simulink model "MCity_cs_withAEBSBlock"  (R2017a)
settings: Solver=ode5  StartTime=0.0  StopTime=3.95  FixedStep=1/200  RelTol=1e-3
PreLoadFcn:
  | check_NUTS_defined;
  | 
  | assignin('base',['model_closed_' bdroot],false);
InitFcn:
  | PreScanExperimentInitFcn(bdroot)
StopFcn:
  | PreScanExperimentStopFcn(bdroot)
model workspace (MAT data in the model file):
  mbox_table : struct (value not decoded)
  model_closed = 0
  sim_status = 0
values from neighbouring files (symbols this model uses):
  d_offset = -18.15    [monocityTestLeftTurn.mat]    (also in simulation_leftTurn_PreScan.m = dl/vl*vh - 43 + R)
undefined symbols (not defined in the file or in its folder): DiscIntNeverNeededParam, warningInitialVelocity, x0
libraries: simulink x78, PreScanSimulinkLibrary x14, simulink_extras x10, PreScanUsefulBlocks x4
(part 12 of 12)

== matlab function MCity_cs_withAEBSBlock/BMW_Z3_1/Subsystem/PreBraking Model/Straight road segment/Relative velocity1/Translation ==
  data: v input; xpd input; xp_dot output; TISdet parameter
function xp_dot = trans(v, xpd, TISdet)
%#codegen
%Translation of the value

xp_dot = xpd;
for i = 1 : TISdet(1)
    if xpd(i) == v
        xp_dot(i) = 0;
    end
end
end

== matlab function MCity_cs_withAEBSBlock/BMW_Z3_1/Subsystem/PreBraking Model/Straight road segment/Relative velocity1/Embedded MATLAB Function1 ==
  settings: updateMethod=DISCRETE
  data: r input; yp2 output; yp1 input; K1 input; K2 output; TISdet parameter; TISMaxRange parameter
function [yp2, K2] = modif(r, yp1, K1, TISdet, TISMaxRange)
%#codegen
% Interpolating yp value.

K2 = K1;
yp2 = yp1;

d = 50;

% Adding point
for i = 1 : TISdet(1)
   if r(i) ~= TISMaxRange(1)
      K2(i,1:d-1) = K2(i,2:d);
      K2(i,d) = yp1(i);
   end
end

% Choosing what to take
for i = 1 : TISdet(1)
    s = 0;
    suma = 0;
    for j = 1 : 50
        if K2(i,j) ~= 0
            suma = suma + K2(i,j);
            s = s + 1;
        end
    end
    yp2(i) = suma/s;
end

% Returning, if object is not detected
for i = 1: TISdet(1)
    if r(i) == TISMaxRange(1) && yp1(i) == 0
        K2(i,:,:) = zeros(d,1);
        yp2(i) = 0;
    end    
end

== matlab function MCity_cs_withAEBSBlock/Audi_A8_1/PathFollower_Preview_1/LateralController/Calculate delta steering error/eml_delta_steering_error ==
  data: v_x_vehicle input; v_x_vehicle_Min input; t_Preview_LatCtrl input; delta_steeringwheeltotal output; v_y_vehicle input; yawrate_vehicle input; CorneringStiffness_Tyres_Front input; CorneringStiffness_Tyres_Rear input; m_vehicle_total input; inertia_z_vehicle_total input; e_Lat input size=10; Pos_x_CoG_Vehicle input; wheelbase input; RefreshCounter parameter
function delta_steeringwheeltotal = eml_delta_steering_error(v_x_vehicle,v_x_vehicle_Min,t_Preview_LatCtrl,v_y_vehicle,yawrate_vehicle,CorneringStiffness_Tyres_Front,CorneringStiffness_Tyres_Rear,m_vehicle_total,inertia_z_vehicle_total,e_Lat,Pos_x_CoG_Vehicle,wheelbase,RefreshCounter)

delta_steeringwheeltotal = emlfcn_delta_steering_error(v_x_vehicle,v_x_vehicle_Min,t_Preview_LatCtrl,v_y_vehicle,yawrate_vehicle,CorneringStiffness_Tyres_Front,CorneringStiffness_Tyres_Rear,m_vehicle_total,inertia_z_vehicle_total,e_Lat,Pos_x_CoG_Vehicle,wheelbase,RefreshCounter);

% end function

== matlab function MCity_cs_withAEBSBlock/BMW_Z3_1/Subsystem/PreBraking Model/Straight road segment/Relative velocity2/Embedded MATLAB Function1 ==
  data: r input; yp2 output; yp1 input; K1 input; K2 output; TISdet parameter; TISMaxRange parameter
function [yp2, K2] = modif(r, yp1, K1, TISdet, TISMaxRange)
%#codegen
% Interpolating yp value.

K2 = K1;
yp2 = yp1;

d = 50;

% Adding point
for i = 1 : TISdet(2)
   if r(i) ~= 5*TISMaxRange(2) 
      K2(i,1:d-1) = K2(i,2:d);
      K2(i,d) = yp1(i);
   end
end

% Choosing what to take
for i = 1 : TISdet(2)
    s = 0;
    suma = 0;
    for j = 1 : 50
        if K2(i,j) ~= 0
            suma = suma + K2(i,j);
            s = s + 1;
        end
    end
    yp2(i) = suma/s;
end

% Returning, if object is not detected
for i = 1: TISdet(2)
    if r(i) == 30 && yp1(i) == 0
        K2(i,:,:) = zeros(d,1);
        yp2(i) = 0;
    end    
end

== matlab function MCity_cs_withAEBSBlock/BMW_Z3_1/Subsystem/PreBraking Model/Straight road segment/Relative velocity2/Translation ==
  data: v input; xpd input; xp_dot output; TISdet parameter
function xp_dot = trans(v, xpd, TISdet)
%#codegen
%Translation of the value

xp_dot = xpd;
for i = 1 : TISdet(2)
    if xpd(i) == v
        xp_dot(i) =0;
    end
end
end

== matlab function MCity_cs_withAEBSBlock/BMW_Z3_1/Subsystem/PreBraking Model/TIS1sorting_fun/Embedded MATLAB Function ==
  data: range input; indx input; RANGE output; TISdet parameter
function RANGE = dis(range, indx, TISdet)
%#codegen

RANGE = zeros(TISdet(1),1);
for i = 1 : length(indx)
    if indx(i) ~= 0
        RANGE(i) = range(indx(i));
    else
        RANGE(i) = 0;
    end
end

== matlab function MCity_cs_withAEBSBlock/BMW_Z3_1/Subsystem/PreBraking Model/Straight road segment/THETA Derivative1/Deriv correction ==
  data: th input; thp input; thd input; th_dot output; TISdet parameter
function th_dot = stopping(th, thp, thd, TISdet)
%#codegen
% Stopping if nothing is detected.

th_dot = thd;
for i = 1 : TISdet(2)
    if (th(i)==0 && thp(i)~=0) || (th(i)~=0 && thp(i)==0)
        th_dot(i) = 0;
    end
end
end

== matlab function MCity_cs_withAEBSBlock/BMW_Z3_1/Subsystem/PreBraking Model/Straight road segment/THETA Derivative2/Deriv correction ==
  data: th input; thp input; thd input; th_dot output; TISdet parameter
function th_dot = stopping(th, thp, thd, TISdet)
%#codegen
% Stopping if nothing is detected.

th_dot = thd;
for i = 1 : TISdet(1)
    if (th(i)==0 && thp(i)~=0) || (th(i)~=0 && thp(i)==0)
        th_dot(i) = 0;
    end
end
end

== matlab function MCity_cs_withAEBSBlock/BMW_Z3_1/Subsystem/PreBraking Model/Straight road segment/THETA Derivative2/Theta extrapolation ==
  data: r input; th1 input; th2 output; thd input; time input; K1 input; K2 output; TISdet parameter; TISMaxRange parameter
function [th2, K2] = modif(r, th1, thd, time, K1, TISdet, TISMaxRange)
%#codegen
% Interpolating theta value.

K2 = K1;
th2 = th1;

d = 10;

% Finding points used in interpolation/extrapolation.
for i = 1 : TISdet(1)
    if thd(i) ~= 0
        K2(i,1:d-1,:) = K2(i,2:d,:);
        K2(i,  d,1) = time;
        K2(i,  d,2) = th1(i);
    end
end

% Extrapolation
for i = 1 : TISdet(1)
    j = 1;
    while j < d+1 && K2(i,j,1) == 0
        j = j + 1;
    end
    
    if j > d-2
        th2(i) = th1(i);
    else
        th2(i) = interp1(K2(i,d-2:d,1),K2(i,d-2:d,2),time,'linear','extrap');
    end
end

% Returning, if object is not detected
for i = 1: TISdet(1)
    if r(i) == TISMaxRange(1) && th1(i) == 0
        K2(i,:,:) = zeros(d,2);
        th2(i) = 0;
    end    
end

end

== matlab function MCity_cs_withAEBSBlock/BMW_Z3_1/Subsystem/PreBraking Model/Straight road segment/THETA Derivative1/Theta extrapolation ==
  data: r input; th1 input; th2 output; thd input; time input; K1 input; K2 output; TISdet parameter; TISMaxRange parameter
function [th2, K2] = modif(r, th1, thd, time, K1, TISdet, TISMaxRange)
%#codegen
% Interpolating theta value.

K2 = K1;
th2 = th1;

d = 10;

% Finding points used in interpolation/extrapolation.
for i = 1 : TISdet(2)
    if thd(i) ~= 0
        K2(i,1:d-1,:) = K2(i,2:d,:);
        K2(i,  d,1) = time;
        K2(i,  d,2) = th1(i);
    end
end

% Extrapolation
for i = 1 : TISdet(2)
    j = 1;
    while j < d+1 && K2(i,j,1) == 0
        j = j + 1;
    end
    
    if j > d-2
        th2(i) = th1(i);
    else
        th2(i) = interp1(K2(i,d-2:d,1),K2(i,d-2:d,2),time,'linear','extrap');
    end
end

% Returning, if object is not detected
for i = 1: TISdet(2)
    if r(i) == 5*TISMaxRange(2) && th1(i) == 0
        K2(i,:,:) = zeros(d,2);
        th2(i) = 0;
    end    
end

end

== matlab function MCity_cs_withAEBSBlock/BMW_Z3_1/Subsystem/PreBraking Model/Bend road segment/T2.6/median filter/median function ==
  data: u input; y output; TISdet parameter
function y = fcn(u, TISdet)
%#codegen


nr = 1;
y = zeros(TISdet(nr),1,'int16');

for kk = 1 : TISdet(nr)
    z = 0;
    w = 0;
    for ii = 0 : 2
        if u(TISdet(nr)*ii+kk) == true
            w = w + 1;
        else
            z = z + 1;
        end
    end
    
    if w > z
        y(kk) = int16(1);
    end
end

end

== matlab function MCity_cs_withAEBSBlock/BMW_Z3_1/Subsystem/PreBraking Model/Bend road segment/T1.6/median filter/median function ==
  data: u input; y output; TISdet parameter
function y = fcn(u, TISdet)
%#codegen


nr = 1;
y = zeros(TISdet(nr),1,'int16');

for kk = 1 : TISdet(nr)
    z = 0;
    w = 0;
    for ii = 0 : 2
        if u(TISdet(nr)*ii+kk) == true
            w = w + 1;
        else
            z = z + 1;
        end
    end
    
    if w > z
        y(kk) = int16(1);
    end
end

end

== matlab function MCity_cs_withAEBSBlock/BMW_Z3_1/Subsystem/PreBraking Model/Straight road segment/T1.6/median filter/median function ==
  data: u input; y output; TISdet parameter
function y = fcn(u, TISdet)
%#codegen


nr = 1;
y = zeros(TISdet(nr),1,'int16');

for kk = 1 : TISdet(nr)
    z = 0;
    w = 0;
    for ii = 0 : 2
        if u(TISdet(nr)*ii+kk) == true
            w = w + 1;
        else
            z = z + 1;
        end
    end
    
    if w > z
        y(kk) = int16(1);
    end
end

end

== matlab function MCity_cs_withAEBSBlock/BMW_Z3_1/Subsystem/PreBraking Model/Straight road segment/T2.6/median filter/median function ==
  data: u input; y output; TISdet parameter
function y = fcn(u, TISdet)
%#codegen


nr = 1;
y = zeros(TISdet(nr),1,'int16');

for kk = 1 : TISdet(nr)
    z = 0;
    w = 0;
    for ii = 0 : 2
        if u(TISdet(nr)*ii+kk) == true
            w = w + 1;
        else
            z = z + 1;
        end
    end
    
    if w > z
        y(kk) = int16(1);
    end
end

end

== matlab function MCity_cs_withAEBSBlock/BMW_Z3_1/Subsystem/PreBraking Model/TIS1sorting_fun/Embedded MATLAB Function1 ==
  data: indx input; THETA output; theta input; TISdet parameter
function THETA = ang(indx, theta, TISdet)
%#codegen

THETA = zeros(TISdet(1),1);
for i = 1 : length(indx)
    if indx(i) ~= 0
        THETA(i) = theta(indx(i));
    else
        THETA(i) = 0;
    end
end

== matlab function MCity_cs_withAEBSBlock/BMW_Z3_1/Subsystem/PreBraking Model/TIS1sorting_fun/Embedded MATLAB Function2 ==
  data: indx input; RANGEDOT output; rangedot input; TISdet parameter
function RANGEDOT = vel(indx, rangedot, TISdet)
%#codegen

RANGEDOT = zeros(TISdet(1),1);
for i = 1 : length(indx)
    if indx(i) ~= 0
        RANGEDOT(i) = rangedot(indx(i));
    else
        RANGEDOT(i) = 0;
    end
end

== matlab function MCity_cs_withAEBSBlock/BMW_Z3_1/Subsystem/PreBraking Model/TIS1sorting_fun/MATLAB Function ==
  data: indxp input; indx output; range input; TISdet parameter
function indx = sorts(indxp, range, TISdet)
%#codegen

size = TISdet(1);

indx = indxp;

for i = 1 : size
    if ( indx(i) ~= 0 ) && ( range(i) == 0)
        indx(i) = 0;
    end
end

for i = 1 : size
    if indx(i) ~= 0
        range(i) = 0;
    end
end

for i = 1 : size
    if range(i) ~= 0
       j = 1;
       while( indx(j) )
           j = j + 1;
       end
       if j ~= size
           indx(j) = i;
       end
    end
end
indx = round(indx);
end

== matlab function MCity_cs_withAEBSBlock/BMW_Z3_1/Subsystem/PreBraking Model/TIS2sorting_fun/Embedded MATLAB Function ==
  data: range input; indx input; RANGE output; TISdet parameter
function RANGE = dis(range, indx, TISdet)
%#codegen

RANGE = zeros(TISdet(2),1);
for i = 1 : length(indx)
    if indx(i) ~= 0
        RANGE(i) = range(indx(i));
    else
        RANGE(i) = 0;
    end
end

== matlab function MCity_cs_withAEBSBlock/BMW_Z3_1/Subsystem/PreBraking Model/TIS2sorting_fun/Embedded MATLAB Function1 ==
  data: indx input; THETA output; theta input; TISdet parameter
function THETA = ang(indx, theta, TISdet)
%#codegen

THETA = zeros(TISdet(2),1);
for i = 1 : length(indx)
    if indx(i) ~= 0
        THETA(i) = theta(indx(i));
    else
        THETA(i) = 0;
    end
end

== matlab function MCity_cs_withAEBSBlock/BMW_Z3_1/Subsystem/PreBraking Model/TIS2sorting_fun/Embedded MATLAB Function2 ==
  data: indx input; RANGEDOT output; rangedot input; TISdet parameter
function RANGEDOT = vel(indx, rangedot, TISdet)
%#codegen

RANGEDOT = zeros(TISdet(2),1);
for i = 1 : length(indx)
    if indx(i) ~= 0
        RANGEDOT(i) = rangedot(indx(i));
    else
        RANGEDOT(i) = 0;
    end
end

== matlab function MCity_cs_withAEBSBlock/BMW_Z3_1/Subsystem/PreBraking Model/TIS2sorting_fun/MATLAB Function ==
  data: indxp input; indx output; range input; TISdet parameter
function indx = sorts(indxp, range, TISdet)
%#codegen

size = TISdet(2);

indx = indxp;

for i = 1 : size
    if ( indx(i) ~= 0 ) && ( range(i) == 0)
        indx(i) = 0;
    end
end

for i = 1 : size
    if indx(i) ~= 0
        range(i) = 0;
    end
end

for i = 1 : size
    if range(i) ~= 0
       j = 1;
       while( indx(j) )
           j = j + 1;
       end
       if j ~= size
           indx(j) = i;
       end
    end
end
indx = round(indx);
end
